simulink model "my_scara_final"  (R2022b)
settings: Solver=daessc  StartTime=0.0  StopTime=7  FixedStep=0.01  RelTol=1e-3
values from neighbouring files (symbols this model uses):
  B_motor = 1.9099e-4    (= 0.00019099)    [DC_motor_init.m]    (also in LOAD_ROBOT_DATA.m = 0.000678; circular_interp.m = 0.000678; computed_torque_control.m; create_model_tree.m)
  ball_screw_ratio = 2*pi*(2/1)/(10e-2)    (= 125.663706144)    [LOAD_ROBOT_DATA.m]    (also in circular_interp.m; computed_torque_control.m; create_model_tree.m; final_script.m)
  gear_ratio_j1 = 10/1    (= 10)    [LOAD_ROBOT_DATA.m]    (also in circular_interp.m; computed_torque_control.m; create_model_tree.m; final_script.m)
  gear_ratio_j2 = 10/1    (= 10)    [LOAD_ROBOT_DATA.m]    (also in circular_interp.m; computed_torque_control.m; create_model_tree.m; final_script.m)
  J_rotor = 2118.45e-7    (= 0.000211845)    [DC_motor_init.m]    (also in LOAD_ROBOT_DATA.m = 0.0125; circular_interp.m = 0.0125; computed_torque_control.m; create_model_tree.m)
  Ke = 0.08    [DC_motor_init.m]    (also in LOAD_ROBOT_DATA.m = 0.957; circular_interp.m = 0.957; computed_torque_control.m; create_model_tree.m)
  Kt = 0.08    [DC_motor_init.m]    (also in LOAD_ROBOT_DATA.m = 0.957; circular_interp.m = 0.957; computed_torque_control.m; create_model_tree.m)
  L = 0.90e-3    (= 0.0009)    [DC_motor_init.m]    (also in LOAD_ROBOT_DATA.m = 0.0054; circular_interp.m = 0.0054; computed_torque_control.m; create_model_tree.m)
  R = 0.43    [DC_motor_init.m]    (also in LOAD_ROBOT_DATA.m = 1.45; circular_interp.m = 1.45; computed_torque_control.m; create_model_tree.m)
  s = tf('s')    [stability_analysis.m]
  upper_sat_voltage = 30    [DC_motor_init.m]    (also in LOAD_ROBOT_DATA.m; circular_interp.m; computed_torque_control.m; create_model_tree.m)
  upper_torque_limit = 4    [DC_motor_init.m]    (also in LOAD_ROBOT_DATA.m; circular_interp.m; computed_torque_control.m = 40; create_model_tree.m)
undefined symbols (not defined in the file or in its folder): smiData, X, Y, Z
libraries: sm_lib x33, nesl_utility x10, robotmaniplib x3, slpidlib x3, robotcorelib x1
(part 2 of 2)

== system my_scara_final/ROBOT/LINK 0/khau0_base_support_1_RIGID ==
  ReferenceFrame : sm_lib/Frames and Transforms/Reference Frame
  Solid : sm_lib/Body Elements/File Solid  ExtGeomFileName=khau0_base_support_Default_sldprt.STEP  UnitType=FromFile  ExtGeomFileUnits=m  StepReaderType=HEX  ExportConvexHullGeometry=off  InertiaType=Custom  Mass=smiData.Solid(6).mass  MassUnits=kg  CenterOfMass=smiData.Solid(6).CoM  CenterOfMassUnits=mm  MomentsOfInertia=smiData.Solid(6).MoI  MomentsOfInertiaUnits=kg*mm^2  ProductsOfInertia=smiData.Solid(6).PoI  ProductsOfInertiaUnits=kg*mm^2  BasedOnType=DensityFromFile  Density=1000  DensityUnits=kg/m^3  DoExposeReferenceFrame=on  SerializedFrames=<Frames/>  GraphicType=FromGeometry  MarkerShape=Sphere  MarkerSize=10  GraphicVisPropType=SimpleVisualProperties  GraphicDiffuseColor=smiData.Solid(6).color  GraphicSpecularColor=[0.5 0.5 0.5 1.0]  GraphicAmbientColor=[0.15 0.15 0.15 1.0]  GraphicEmissiveColor=[0.0 0.0 0.0 1.0]  GraphicShininess=75  GraphicOpacity=smiData.Solid(6).opacity
  F : PMIOPort  Side=Left
  connections:
  F/RConn1 -- ReferenceFrame/RConn1 -- Solid/RConn1
